simulink model "rule1"  (Simulink 9.1)
settings: Solver=FixedStepDiscrete  StartTime=0  StopTime=31.96  FixedStep=0.01  RelTol=1e-3
settings Model: Creator=Hengyi  LastModifiedBy=Hengyi
settings DataIOCC: SaveFormat=StructureWithTime  SaveOutput=off  SaveTime=off
settings OptimizationCC: LifeSpan=auto
settings DebuggingCC: UnderspecifiedInitializationDetection=Simplified  MergeDetectMultiDrivingBlocksExec=error  SFUnexpectedBacktrackingDiag=error  SFNoUnconditionalDefaultTransitionDiag=error  SFExecutionAtInitializationDiag=warning
settings HardwareCC: ProdBitPerPointer=64  ProdBitPerSizeT=64  ProdBitPerPtrDiffT=64  ProdLargestAtomicFloat=Float  ProdIntDivRoundTo=Zero  ProdEndianess=LittleEndian  ProdWordSize=64  ProdHWDeviceType=Intel->x86-64 (Windows64)
settings ModelReferenceCC: PropagateSignalLabelsOutOfModel=on
settings CodeAppCC: StateflowObjectComments=off
settings GRTTargetCC: TargetLangStandard=C99 (ISO)  CombineOutputUpdateFcns=on  GRTInterface=off
settings ConfigComp: CovMetricSettings=dwe  CovHtmlReporting=off  CovSaveCumulativeToWorkspaceVar=off  CovSaveSingleToWorkspaceVar=off  CovExternalEMLEnable=on

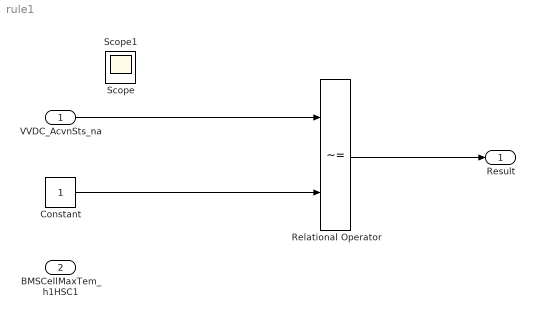
== system rule1 ==
  VVDC_AcvnSts_na : Inport  OutDataTypeStr=double
  BMSCellMaxTem_h1HSC1 : Inport  Port=2  OutDataTypeStr=double
  Constant : Constant
  Relational Operator : RelationalOperator  Operator=~=  OutDataTypeStr=boolean  RndMeth=Simplest
  Result : Outport
  Scope : Scope
  Scope1 : Scope
  wires:
  VVDC_AcvnSts_na/1 -> Relational Operator/1
  Relational Operator/1 -> Result/1
  Constant/1 -> Relational Operator/2
